simulink model "DIL_2023a"  (R2023b)
settings: Solver=VariableStepAuto  StartTime=0.0  StopTime=12  RelTol=1e-2
values from neighbouring files (symbols this model uses):
  s0 = load("s0.mat").s1(1:22)    [DIL_matlab.m]    (also in setup.m = load("s0.mat").s1(1:18)')
settings Model: SimulationMode=accelerator  Creator=Inver  LastModifiedBy=Inver
settings SolverCC: SolverJacobianMethodControl=FullAnalytical  DaesscMode=Robust  ZeroCrossAlgorithm=Adaptive

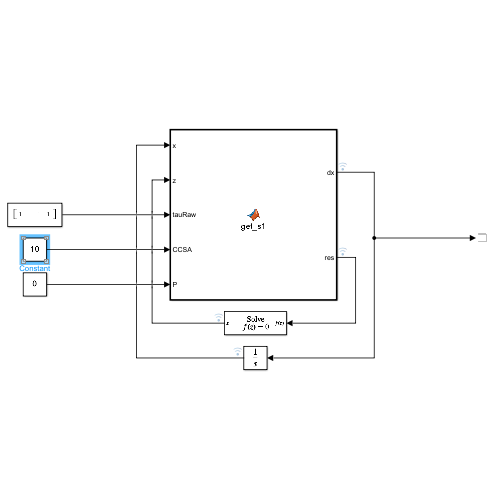
[thumbnail: Simulink's stored preview of the top-level diagram]
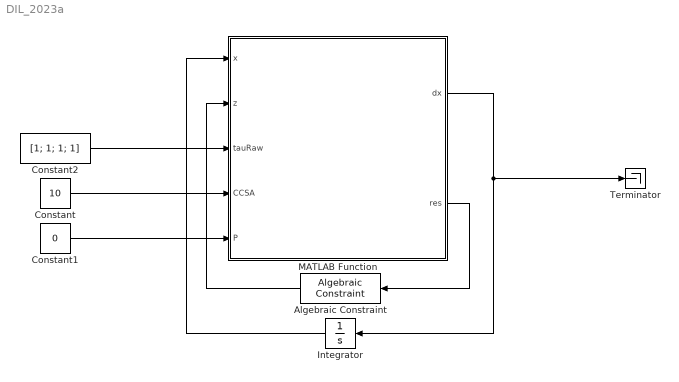
== system DIL_2023a ==
  Algebraic Constraint : AlgebraicConstraint  Tolerance=1e-6  InitialGuess=zeros(4, 1)
  Constant : Constant  Value=10
  Constant1 : Constant  Value=0
  Constant2 : Constant  Value=[1; 1; 1; 1]
  Integrator : Integrator  InitialCondition=s0
  MATLAB Function : MATLAB Function  TreatAsAtomicUnit=on
  Terminator : Terminator
  wires:
  MATLAB Function/1(dx) -> Integrator/1, Terminator/1
  Integrator/1 -> MATLAB Function/1(x)
  Constant/1 -> MATLAB Function/4(CCSA)
  Constant1/1 -> MATLAB Function/5(P)
  Constant2/1 -> MATLAB Function/3(tauRaw)
  MATLAB Function/2(res) -> Algebraic Constraint/1
  Algebraic Constraint/1 -> MATLAB Function/2(z)

== matlab function DIL_2023a/MATLAB Function ==
  data: x input; z input; dx output; tauRaw input; CCSA input; P input; varCAR parameter; res output
function [dx, res] = get_s1(x, z, tauRaw, CCSA, P, varCAR)
    s = [x; z];

    [xS, yS, zS, dxS, dyS, dzS, xT, yT, zT] = vehicle_suspension(s, varCAR);
    [SA, w] = vehicle_slip(s, CCSA, xT, yT, varCAR);
    [sum_Fxa, sum_Fya, sum_Fza, sum_Mx, sum_My, sum_Mz, res_torque] = vehicle_forces(s, CCSA, P, w, SA, xT, yT, zS, dzS, tauRaw, varCAR);
    derivatives = vehicle_dynamics(s, sum_Fxa, sum_Fya, sum_Fza, sum_Mx, sum_My, sum_Mz, res_torque, varCAR);
    [dVb, dAs, dT] = vehicle_powertrain(s, tauRaw, w, varCAR);

    dx = [derivatives; dVb; dAs; dT];
    res = res_torque;

    ds = [dx; res];

    if sum(isnan(ds)) || sum(isinf(ds))
        stop = 1;
    end
end
